simulink model "CSE1_CV3_1Straight"  (Simulink 7.3)
settings: Solver=ode4  StartTime=0.0  StopTime=inf  FixedStep=0.1  RelTol=1e-3
undefined symbols (not defined in the file or in its folder): eta1_0_real, v1_0_real, velocitySatValues1
libraries: simulink x68, dspmtrx3 x24, simulink_extras x23, marine_gnc x5, dspindex x5, dspinverses x4
(part 2 of 6)

== system CSE1_CV3_1Straight/Plants/CSE1 ==
  Thurster setting : Inport
  Enable : EnablePort  StatesWhenEnabling=reset
  Bow Thruster : Subsystem
  Demux : Demux  Outputs=7
  "Voith Schneider Propeller " : Subsystem
  wires:
  Thurster setting/1 -> Demux/1
  Demux/1 -> "Voith Schneider Propeller "/1(Port VSP y u_1)
  Demux/2 -> "Voith Schneider Propeller "/2(Port VSP x u_2)
  Demux/3 -> "Voith Schneider Propeller "/3(Starboard VSP y u_3)
  Demux/4 -> "Voith Schneider Propeller "/4(Starboard VSP x u_4)
  Demux/7 -> "Voith Schneider Propeller "/5(VSP Speed)
  Demux/5 -> Bow Thruster/1(Bow Thruster Direction u_5)
  Demux/6 -> Bow Thruster/2(Bow Thruster Power)

== system CSE1_CV3_1Straight/Plants/Linear Simulator ==
  tau : Inport
  Enable : EnablePort  StatesWhenEnabling=reset
  Demux1 : Demux  Outputs=3
  Demux2 : Demux  Outputs=3
  Demux3 : Demux  Outputs=3
  Linear Vessel Dynamics : Subsystem
  Mux1 : Mux  Inputs=3
  Mux2 : Mux  Inputs=3
  Mux3 : Mux  Inputs=3
  eta_surge_hil : Gain  ParameterDataType=fixdt(1, 16)  ParameterScaling=2^0  OutDataType=fixdt(1, 16)  OutScaling=2^0
  eta_sway_hil : Gain  ParameterDataType=fixdt(1, 16)  ParameterScaling=2^0  OutDataType=fixdt(1, 16)  OutScaling=2^0
  eta_yaw_hil : Gain  ParameterDataType=fixdt(1, 16)  ParameterScaling=2^0  OutDataType=fixdt(1, 16)  OutScaling=2^0
  etadot : Terminator
  etadot_surge_hil : Gain  ParameterDataType=fixdt(1, 16)  ParameterScaling=2^0  OutDataType=fixdt(1, 16)  OutScaling=2^0
  etadot_sway_hil : Gain  ParameterDataType=fixdt(1, 16)  ParameterScaling=2^0  OutDataType=fixdt(1, 16)  OutScaling=2^0
  etadot_yaw_hil : Gain  ParameterDataType=fixdt(1, 16)  ParameterScaling=2^0  OutDataType=fixdt(1, 16)  OutScaling=2^0
  nu_surge_hil : Gain  ParameterDataType=fixdt(1, 16)  ParameterScaling=2^0  OutDataType=fixdt(1, 16)  OutScaling=2^0
  nu_sway_hil : Gain  ParameterDataType=fixdt(1, 16)  ParameterScaling=2^0  OutDataType=fixdt(1, 16)  OutScaling=2^0
  nu_yaw_hil : Gain  ParameterDataType=fixdt(1, 16)  ParameterScaling=2^0  OutDataType=fixdt(1, 16)  OutScaling=2^0
  eta_hil : Outport
  nu_hil : Outport  Port=2
  wires:
  nu_yaw_hil/1 -> Mux1/3
  nu_sway_hil/1 -> Mux1/2
  nu_surge_hil/1 -> Mux1/1
  Demux2/3 -> nu_yaw_hil/1
  Demux2/2 -> nu_sway_hil/1
  Demux2/1 -> nu_surge_hil/1
  eta_sway_hil/1 -> Mux3/2
  eta_yaw_hil/1 -> Mux3/3
  eta_surge_hil/1 -> Mux3/1
  Demux1/3 -> eta_yaw_hil/1
  Demux1/2 -> eta_sway_hil/1
  Demux1/1 -> eta_surge_hil/1
  Linear Vessel Dynamics/1(eta) -> Demux1/1
  Linear Vessel Dynamics/2(nu) -> Demux2/1
  Mux1/1 -> nu_hil/1
  Mux3/1 -> eta_hil/1
  etadot_sway_hil/1 -> Mux2/2
  etadot_yaw_hil/1 -> Mux2/3
  etadot_surge_hil/1 -> Mux2/1
  Demux3/3 -> etadot_yaw_hil/1
  Demux3/2 -> etadot_sway_hil/1
  Demux3/1 -> etadot_surge_hil/1
  Linear Vessel Dynamics/3(etadot) -> Demux3/1
  Mux2/1 -> etadot/1
  tau/1 -> Linear Vessel Dynamics/1(tau)

== system CSE1_CV3_1Straight/Plants/saturation ==
  tau : Inport  OutDataType=sfix(16)  OutScaling=2^0
  Demux : Demux  Outputs=3
  Mux1 : Mux  Inputs=3
  Saturation : Saturate  UpperLimit=3  LowerLimit=-2.6
  Saturation1 : Saturate  UpperLimit=3  LowerLimit=-3.5
  Saturation2 : Saturate  UpperLimit=1.6  LowerLimit=-1.5
  plant tau_surge : Gain  ParameterDataType=fixdt(1, 16)  ParameterScaling=2^0  OutDataType=fixdt(1, 16)  OutScaling=2^0
  plant tau_sway : Gain  ParameterDataType=fixdt(1, 16)  ParameterScaling=2^0  OutDataType=fixdt(1, 16)  OutScaling=2^0
  plant tau_yaw : Gain  ParameterDataType=fixdt(1, 16)  ParameterScaling=2^0  OutDataType=fixdt(1, 16)  OutScaling=2^0
  sat_tau : Outport  OutDataType=sfix(16)  OutScaling=2^0
  wires:
  Saturation2/1 -> plant tau_yaw/1
  Saturation1/1 -> plant tau_sway/1
  Saturation/1 -> plant tau_surge/1
  Demux/3 -> Saturation2/1
  Demux/2 -> Saturation1/1
  Demux/1 -> Saturation/1
  tau/1 -> Demux/1
  Mux1/1 -> sat_tau/1
  plant tau_surge/1 -> Mux1/1
  plant tau_sway/1 -> Mux1/2
  plant tau_yaw/1 -> Mux1/3

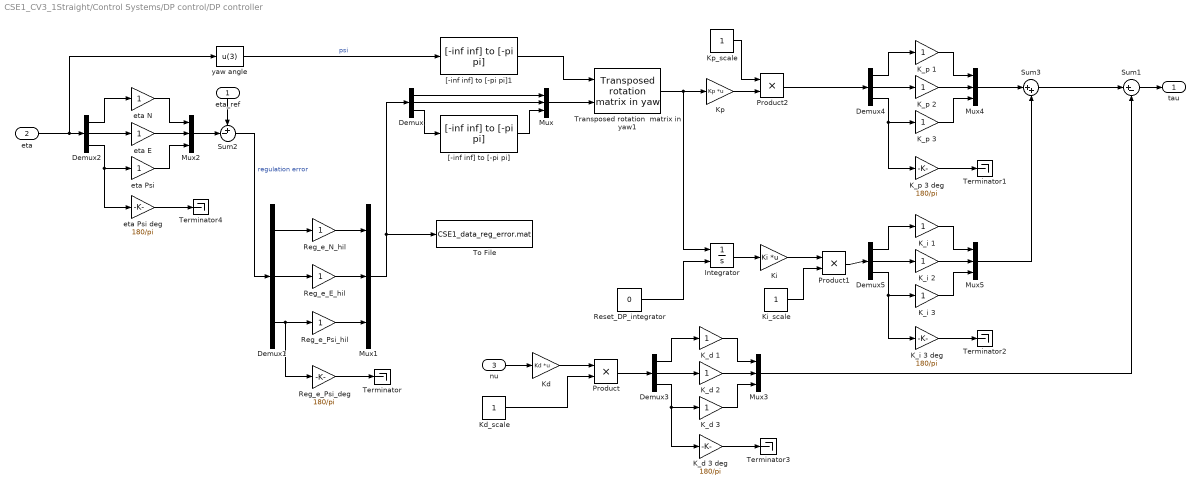
== system CSE1_CV3_1Straight/Control Systems/DP control/DP controller ==
  eta_ref : Inport
  eta : Inport  Port=2
  nu : Inport  Port=3
  Demux{,1..5} (6 alike) : Demux  Outputs=3
  Integrator : Integrator  ExternalReset=level
  K_d 1 : Gain  ParameterDataType=fixdt(1, 16)  ParameterScaling=2^0  OutDataType=fixdt(1, 16)  OutScaling=2^0
  K_d 2 : Gain  ParameterDataType=fixdt(1, 16)  ParameterScaling=2^0  OutDataType=fixdt(1, 16)  OutScaling=2^0
  K_d 3 : Gain  ParameterDataType=fixdt(1, 16)  ParameterScaling=2^0  OutDataType=fixdt(1, 16)  OutScaling=2^0
  K_d 3 deg : Gain  Gain=180/pi  ParameterDataType=fixdt(1, 16)  ParameterScaling=2^0  OutDataType=fixdt(1, 16)  OutScaling=2^0
  K_i 1 : Gain  ParameterDataType=fixdt(1, 16)  ParameterScaling=2^0  OutDataType=fixdt(1, 16)  OutScaling=2^0
  K_i 2 : Gain  ParameterDataType=fixdt(1, 16)  ParameterScaling=2^0  OutDataType=fixdt(1, 16)  OutScaling=2^0
  K_i 3 : Gain  ParameterDataType=fixdt(1, 16)  ParameterScaling=2^0  OutDataType=fixdt(1, 16)  OutScaling=2^0
  K_i 3 deg : Gain  Gain=180/pi  ParameterDataType=fixdt(1, 16)  ParameterScaling=2^0  OutDataType=fixdt(1, 16)  OutScaling=2^0
  K_p 1 : Gain  ParameterDataType=fixdt(1, 16)  ParameterScaling=2^0  OutDataType=fixdt(1, 16)  OutScaling=2^0
  K_p 2 : Gain  ParameterDataType=fixdt(1, 16)  ParameterScaling=2^0  OutDataType=fixdt(1, 16)  OutScaling=2^0
  K_p 3 : Gain  ParameterDataType=fixdt(1, 16)  ParameterScaling=2^0  OutDataType=fixdt(1, 16)  OutScaling=2^0
  K_p 3 deg : Gain  Gain=180/pi  ParameterDataType=fixdt(1, 16)  ParameterScaling=2^0  OutDataType=fixdt(1, 16)  OutScaling=2^0
  Kd : Gain  Gain=Kd  Multiplication=Matrix(K*u)  SaturateOnIntegerOverflow=on  OutDataTypeStr=Inherit: Same as input  ParamDataTypeStr=Inherit: Same as input
  Kd_scale : Constant
  Ki : Gain  Gain=Ki  Multiplication=Matrix(K*u)  SaturateOnIntegerOverflow=on  OutDataTypeStr=Inherit: Same as input  ParamDataTypeStr=Inherit: Same as input
  Ki_scale : Constant
  Kp : Gain  Gain=Kp  Multiplication=Matrix(K*u)  SaturateOnIntegerOverflow=on  OutDataTypeStr=Inherit: Same as input  ParamDataTypeStr=Inherit: Same as input
  Kp_scale : Constant
  Mux{,1..5} (6 alike) : Mux  Inputs=3
  Product : Product  RndMeth=Zero
  Product1 : Product  RndMeth=Zero
  Product2 : Product  RndMeth=Zero
  Reg_e_E_hil : Gain
  Reg_e_N_hil : Gain
  Reg_e_Psi_deg : Gain  Gain=180/pi  ParameterDataType=fixdt(1, 16)  ParameterScaling=2^0  OutDataType=fixdt(1, 16)  OutScaling=2^0
  Reg_e_Psi_hil : Gain
  Reset_DP_integrator : Constant  Value=0
  Sum1 : Sum  Inputs=|+-  SaturateOnIntegerOverflow=on  InputSameDT=on  OutDataTypeStr=Inherit: Same as first input
  Sum2 : Sum  Inputs=+-|  SaturateOnIntegerOverflow=on  InputSameDT=on  OutDataTypeStr=Inherit: Same as first input
  Sum3 : Sum  Inputs=|++  SaturateOnIntegerOverflow=on  InputSameDT=on  OutDataTypeStr=Inherit: Same as first input
  Terminator{,1..4} (5 alike) : Terminator
  To File : ToFile  Filename=CSE1_data_reg_error.mat  MatrixName=cse1_data_reg_error
  Transposed rotation  matrix in yaw1 : marine_gnc/Models/ Kinematics/Transposed rotation  matrix in yaw  SystemSampleTime=-1
  "[-inf inf] to [-pi pi]" : marine_gnc/Utilities/Math Operations/[-inf inf] to [-pi pi]  SystemSampleTime=-1
  "[-inf inf] to [-pi pi]1" : marine_gnc/Utilities/Math Operations/[-inf inf] to [-pi pi]  SystemSampleTime=-1
  eta E : Gain  ParameterDataType=fixdt(1, 16)  ParameterScaling=2^0  OutDataType=fixdt(1, 16)  OutScaling=2^0
  eta N : Gain  ParameterDataType=fixdt(1, 16)  ParameterScaling=2^0  OutDataType=fixdt(1, 16)  OutScaling=2^0
  eta Psi : Gain  ParameterDataType=fixdt(1, 16)  ParameterScaling=2^0  OutDataType=fixdt(1, 16)  OutScaling=2^0
  eta Psi deg : Gain  Gain=180/pi  ParameterDataType=fixdt(1, 16)  ParameterScaling=2^0  OutDataType=fixdt(1, 16)  OutScaling=2^0
  yaw angle : Fcn  Expr=u(3)
  tau : Outport  InitialOutput=0
  wires:
  Mux/1 -> Transposed rotation  matrix in yaw1/2
  Demux/1 -> Mux/1
  Demux/2 -> Mux/2
  eta_ref/1 -> Sum2/1
  Sum1/1 -> tau/1
  eta/1 -> yaw angle/1, Demux2/1
  Integrator/1 -> Ki/1
  Sum3/1 -> Sum1/1
  Transposed rotation  matrix in yaw1/1 -> Kp/1, Integrator/1
  Demux1/1 -> Reg_e_N_hil/1
  Reg_e_N_hil/1 -> Mux1/1
  Sum2/1 -> Demux1/1  "regulation error"
  Demux1/2 -> Reg_e_E_hil/1
  Reg_e_E_hil/1 -> Mux1/2
  Demux1/3 -> Reg_e_Psi_hil/1, Reg_e_Psi_deg/1
  Reg_e_Psi_hil/1 -> Mux1/3
  Mux1/1 -> Demux/1, To File/1
  nu/1 -> Kd/1
  Kd/1 -> Product/1
  Kd_scale/1 -> Product/2
  Ki/1 -> Product1/1
  Ki_scale/1 -> Product1/2
  Kp/1 -> Product2/2
  Kp_scale/1 -> Product2/1
  Reset_DP_integrator/1 -> Integrator/2
  yaw angle/1 -> "[-inf inf] to [-pi pi]1"/1  "psi"
  "[-inf inf] to [-pi pi]1"/1 -> Transposed rotation  matrix in yaw1/1
  Demux/3 -> "[-inf inf] to [-pi pi]"/1
  "[-inf inf] to [-pi pi]"/1 -> Mux/3
  eta N/1 -> Mux2/1
  eta E/1 -> Mux2/2
  eta Psi/1 -> Mux2/3
  Demux2/1 -> eta N/1
  Demux2/2 -> eta E/1
  Demux2/3 -> eta Psi/1, eta Psi deg/1
  Mux2/1 -> Sum2/2
  K_d 1/1 -> Mux3/1
  K_d 2/1 -> Mux3/2
  K_d 3/1 -> Mux3/3
  Demux3/1 -> K_d 1/1
  Demux3/2 -> K_d 2/1
  Demux3/3 -> K_d 3/1, K_d 3 deg/1
  Product/1 -> Demux3/1
  Mux3/1 -> Sum1/2
  K_p 1/1 -> Mux4/1
  K_p 2/1 -> Mux4/2
  K_p 3/1 -> Mux4/3
  Demux4/1 -> K_p 1/1
  Demux4/2 -> K_p 2/1
  Demux4/3 -> K_p 3/1, K_p 3 deg/1
  Product2/1 -> Demux4/1
  Mux4/1 -> Sum3/1
  K_i 1/1 -> Mux5/1
  K_i 2/1 -> Mux5/2
  K_i 3/1 -> Mux5/3
  Demux5/1 -> K_i 1/1
  Demux5/2 -> K_i 2/1
  Demux5/3 -> K_i 3/1, K_i 3 deg/1
  Product1/1 -> Demux5/1
  Mux5/1 -> Sum3/2
  K_p 3 deg/1 -> Terminator1/1
  K_i 3 deg/1 -> Terminator2/1
  K_d 3 deg/1 -> Terminator3/1
  Reg_e_Psi_deg/1 -> Terminator/1
  eta Psi deg/1 -> Terminator4/1

== system CSE1_CV3_1Straight/Control Systems/DP control/Thruster allocation ==
  tau : Inport
  f_act to u_act : Subsystem
  tau to f_act : Subsystem
  u_act : Outport
  wires:
  tau/1 -> tau to f_act/1(tau)
  tau to f_act/1(f_act) -> f_act to u_act/1(f_act)
  f_act to u_act/1(u_act) -> u_act/1

== system CSE1_CV3_1Straight/Control Systems/LgV design 2/Auxilary functions g_q ==
  f_q : Inport
  psi_los^q : Inport  Port=2
  f_q^q : Inport  Port=3
  psi_los^q^2 : Inport  Port=4
  f_q^s : Inport  Port=5
  psi_los^qs : Inport  Port=6
  f_q^t : Inport  Port=7
  g_q eq : Subsystem
  g_q^q eq : Subsystem
  g_q^s eq : Subsystem
  g_q^t eq : Subsystem
  g_q : Outport
  g_q^t : Outport  Port=2
  g_q^q : Outport  Port=3
  g_q^s : Outport  Port=4
  wires:
  g_q eq/1(g_q) -> g_q/1
  psi_los^q/1 -> g_q eq/2(psi_los^q), g_q^q eq/2(psi_los^q), g_q^s eq/2(psi_los^q), g_q^t eq/1(psi_los^q)
  f_q/1 -> g_q eq/1(f_q), g_q^q eq/1(f_q), g_q^s eq/1(f_q)
  f_q^q/1 -> g_q^q eq/3(f_q^q)
  psi_los^q^2/1 -> g_q^q eq/4(psi_los^q^2)
  g_q^q eq/1(g_q^q) -> g_q^q/1
  g_q^s eq/1(g_q^s) -> g_q^s/1
  f_q^s/1 -> g_q^s eq/3(f_q^s)
  psi_los^qs/1 -> g_q^s eq/4(psi_los^qs)
  g_q^t eq/1(g_q^t) -> g_q^t/1
  f_q^t/1 -> g_q^t eq/2(f_q^t)

== system CSE1_CV3_1Straight/Control Systems/LgV design 2/Auxiliary function g_s ==
  psi_los^sq : Inport
  f_s : Inport  Port=2
  psi_los^s : Inport  Port=3
  f_s^q : Inport  Port=4
  f_s^s : Inport  Port=5
  psi_los^s^2 : Inport  Port=6
  f_s^t : Inport  Port=7
  g_s eq : Subsystem
  g_s^q eq : Subsystem
  g_s^s eq : Subsystem
  g_s^t eq : Subsystem
  g_s^q : Outport
  g_s^s : Outport  Port=2
  g_s^t : Outport  Port=3
  g_s : Outport  Port=4
  wires:
  f_s/1 -> g_s eq/1(f_s), g_s^q eq/1(f_s), g_s^s eq/1(f_s)
  psi_los^s/1 -> g_s eq/2(psi_los^s), g_s^q eq/2(psi_los^s), g_s^s eq/2(psi_los^s), g_s^t eq/1(psi_los^s)
  g_s eq/1(g_s) -> g_s/1
  f_s^q/1 -> g_s^q eq/3(f_s^q)
  psi_los^sq/1 -> g_s^q eq/4(psi_los^sq)
  g_s^q eq/1(g_s^q) -> g_s^q/1
  g_s^s eq/1(g_s^s) -> g_s^s/1
  f_s^s/1 -> g_s^s eq/3(f_s^s)
  psi_los^s^2/1 -> g_s^s eq/4(psi_los^s^2)
  g_s^t eq/1(g_a^t) -> g_s^t/1
  f_s^t/1 -> g_s^t eq/2(f_s^t)

== system CSE1_CV3_1Straight/Control Systems/LgV design 2/Control law ==
  R^T : Inport
  kappa1 : Inport  Port=2
  sigma : Inport  Port=3
  alpha^q : Inport  Port=4
  alpha^s : Inport  Port=5
  nu : Inport  Port=6
  z_2 : Inport  Port=7
  zeta : Inport  Port=8
  omega_q : Inport  Port=9
  K_i : Inport  Port=10
  K_d : Inport  Port=11
  M : Inport  Port=12
  f_q : Inport  Port=13
  f_s : Inport  Port=14
  1 : Constant  OutDataType=fixdt(1, 16)  OutScaling=2^0
  4 : Gain  Gain=4  ParameterDataType=fixdt(1, 16)  ParameterScaling=2^0  OutDataType=fixdt(1, 16)  OutScaling=2^0
  Add1 : Sum  OutDataType=fixdt(1, 16)  OutScaling=2^-10
  Add2 : Sum  OutDataType=fixdt(1, 16)  OutScaling=2^-10
  D_L : Subsystem
  Divide : Product  Inputs=*/  OutDataType=fixdt(1, 16)  OutScaling=2^-10
  Product : Product  Inputs=3  Multiplication=Matrix(*)  OutDataType=fixdt(1, 16)  OutScaling=2^0  RndMeth=Zero
  Product1 : Product  Multiplication=Matrix(*)  OutDataType=fixdt(1, 16)  OutScaling=2^0  RndMeth=Zero
  Product2 : Product  Multiplication=Matrix(*)  OutDataType=fixdt(1, 16)  OutScaling=2^0  RndMeth=Zero
  Product4 : Product  Multiplication=Matrix(*)  OutDataType=fixdt(1, 16)  OutScaling=2^0  RndMeth=Zero
  Product5 : Product  Inputs=3  Multiplication=Matrix(*)  OutDataType=fixdt(1, 16)  OutScaling=2^0  RndMeth=Zero
  Product6 : Product  Inputs=3  Multiplication=Matrix(*)  OutDataType=fixdt(1, 16)  OutScaling=2^0  RndMeth=Zero
  Sum : Sum  Inputs=--++++  OutDataType=fixdt(1, 16)  OutScaling=2^-10
  tau : Outport
  wires:
  Sum/1 -> tau/1
  R^T/1 -> Product/1
  K_i/1 -> Product/2
  zeta/1 -> Product/3
  K_d/1 -> Add1/1
  Divide/1 -> Add1/2
  1/1 -> Divide/1
  kappa1/1 -> 4/1
  4/1 -> Divide/2
  Add1/1 -> Product1/1
  z_2/1 -> Product1/2
  Product1/1 -> Sum/2
  nu/1 -> Product2/2
  D_L/1(D_L) -> Product2/1
  Product2/1 -> Sum/3
  M/1 -> Product4/1, Product5/1, Product6/1
  sigma/1 -> Product4/2
  Product4/1 -> Sum/4
  alpha^q/1 -> Product5/2
  Product5/1 -> Sum/5
  alpha^s/1 -> Product6/2
  f_s/1 -> Product6/3
  Product6/1 -> Sum/6
  omega_q/1 -> Add2/1
  f_q/1 -> Add2/2
  Add2/1 -> Product5/3
  Product/1 -> Sum/1

== system CSE1_CV3_1Straight/Control Systems/LgV design 2/Gamma_q ==
  11 : Inport
  22 : Inport  Port=2
  12 : Constant  Value=0
  21 : Constant  Value=0
  2x2 : Reshape  OutputDimensionality=Customize  OutputDimensions=[2,2]
  Mux : Mux
  Gamma_q : Outport
  wires:
  2x2/1 -> Gamma_q/1
  Mux/1 -> 2x2/1
  11/1 -> Mux/1
  21/1 -> Mux/2
  12/1 -> Mux/3
  22/1 -> Mux/4

== system CSE1_CV3_1Straight/Control Systems/LgV design 2/Integral action state ==
  z_2 : Inport
  R : Inport  Port=2
  Integrator : Integrator  InitialCondition=[0 0 0]'
  Product : Product  Multiplication=Matrix(*)  OutDataType=fixdt(1, 16)  OutScaling=2^0  RndMeth=Zero
  zeta : Outport
  wires:
  R/1 -> Product/1
  z_2/1 -> Product/2
  Integrator/1 -> zeta/1
  Product/1 -> Integrator/1

== system CSE1_CV3_1Straight/Control Systems/LgV design 2/K_d ==
  11 : Inport
  22 : Inport  Port=2
  33 : Inport  Port=3
  {12..13,21,23,31..32} (6 alike) : Constant  Value=0
  3x3 : Reshape  OutputDimensionality=Customize  OutputDimensions=[3,3]
  Mux : Mux  Inputs=9
  K_d : Outport
  wires:
  3x3/1 -> K_d/1
  Mux/1 -> 3x3/1
  11/1 -> Mux/1
  21/1 -> Mux/2
  31/1 -> Mux/3
  12/1 -> Mux/4
  22/1 -> Mux/5
  32/1 -> Mux/6
  13/1 -> Mux/7
  23/1 -> Mux/8
  33/1 -> Mux/9

== system CSE1_CV3_1Straight/Control Systems/LgV design 2/K_i ==
  11 : Inport
  22 : Inport  Port=2
  33 : Inport  Port=3
  {12..13,21,23,31..32} (6 alike) : Constant  Value=0
  3x3 : Reshape  OutputDimensionality=Customize  OutputDimensions=[3,3]
  Mux : Mux  Inputs=9
  K_i : Outport
  wires:
  3x3/1 -> K_i/1
  Mux/1 -> 3x3/1
  11/1 -> Mux/1
  21/1 -> Mux/2
  31/1 -> Mux/3
  12/1 -> Mux/4
  22/1 -> Mux/5
  32/1 -> Mux/6
  13/1 -> Mux/7
  23/1 -> Mux/8
  33/1 -> Mux/9

== system CSE1_CV3_1Straight/Control Systems/LgV design 2/K_p ==
  11 : Inport
  22 : Inport  Port=2
  33 : Inport  Port=3
  {12..13,21,23,31..32} (6 alike) : Constant  Value=0
  Mux : Mux  Inputs=9
  R(psi) : Reshape  OutputDimensionality=Customize  OutputDimensions=[3,3]
  K_p : Outport
  wires:
  R(psi)/1 -> K_p/1
  Mux/1 -> R(psi)/1
  11/1 -> Mux/1
  21/1 -> Mux/2
  31/1 -> Mux/3
  12/1 -> Mux/4
  22/1 -> Mux/5
  32/1 -> Mux/6
  13/1 -> Mux/7
  23/1 -> Mux/8
  33/1 -> Mux/9

== system CSE1_CV3_1Straight/Control Systems/LgV design 2/M ==
  3x3 : Reshape  OutputDimensionality=Customize  OutputDimensions=[3,3]
  I_z : Constant  Value=1.760
  M_{11,22..23,32..33} (5 alike) : Sum  Inputs=+-
  M_{12..13,21,31} (4 alike) : Constant  Value=0
  Mux : Mux  Inputs=9
  N_rdot : Constant  Value=-1.0
  N_vdot : Constant  Value=-0.0
  X_udot : Constant  Value=-2.0
  Y_rdot : Constant  Value=0.0
  Y_vdot : Constant  Value=-10.0
  m : Constant  Value=17.6
  m x_g : Product  RndMeth=Zero
  x_g : Constant  Value=0.03
  M : Outport
  wires:
  3x3/1 -> M/1
  Mux/1 -> 3x3/1
  M_33/1 -> Mux/9
  M_23/1 -> Mux/8
  M_13/1 -> Mux/7
  M_32/1 -> Mux/6
  M_22/1 -> Mux/5
  M_12/1 -> Mux/4
  M_31/1 -> Mux/3
  M_21/1 -> Mux/2
  M_11/1 -> Mux/1
  N_rdot/1 -> M_33/2
  I_z/1 -> M_33/1
  Y_rdot/1 -> M_23/2
  N_vdot/1 -> M_32/2
  m x_g/1 -> M_23/1, M_32/1
  x_g/1 -> m x_g/2
  Y_vdot/1 -> M_22/2
  X_udot/1 -> M_11/2
  m/1 -> m x_g/1, M_22/1, M_11/1

== system CSE1_CV3_1Straight/Control Systems/LgV design 2/R(psi) ==
  psi : Inport
  -1 : Gain  Gain=-1  ParameterDataType=fixdt(1, 16)  ParameterScaling=2^0  OutDataType=fixdt(1, 16)  OutScaling=2^0
  Mux : Mux  Inputs=9
  R(psi) : Reshape  OutputDimensionality=Customize  OutputDimensions=[3,3]
  R11 : Trigonometry  Operator=cos
  R12 : Trigonometry
  R{13,23,31..32} (4 alike) : Constant  Value=0
  R21 : Trigonometry
  R22 : Trigonometry  Operator=cos
  R33 : Constant
  R : Outport
  wires:
  R(psi)/1 -> R/1
  Mux/1 -> R(psi)/1
  psi/1 -> R11/1, R21/1, R12/1, R22/1
  R11/1 -> Mux/1
  R21/1 -> Mux/2
  R31/1 -> Mux/3
  R12/1 -> -1/1
  R22/1 -> Mux/5
  R32/1 -> Mux/6
  R13/1 -> Mux/7
  R33/1 -> Mux/9
  R23/1 -> Mux/8
  -1/1 -> Mux/4

== system CSE1_CV3_1Straight/Control Systems/LgV design 2/S(r) ==
  r : Inport
  Mux : Mux  Inputs=9
  R31 : Constant  Value=0
  S(r) : Reshape  OutputDimensionality=Customize  OutputDimensions=[3,3]
  S{11,13,22..23,32} (5 alike) : Constant  Value=0
  S12 : Gain  ParameterDataType=fixdt(1, 16)  ParameterScaling=2^0  OutDataType=fixdt(1, 16)  OutScaling=2^0
  S33 : Constant
  S : Outport
  wires:
  S(r)/1 -> S/1
  Mux/1 -> S(r)/1
  R31/1 -> Mux/3
  S12/1 -> Mux/4
  S22/1 -> Mux/5
  S32/1 -> Mux/6
  S13/1 -> Mux/7
  S33/1 -> Mux/9
  S23/1 -> Mux/8
  r/1 -> Mux/2, S12/1
  S11/1 -> Mux/1

== system CSE1_CV3_1Straight/Control Systems/LgV design 2/Thruster allocation ==
  tau : Inport
  f_act to u_act : Subsystem
  tau to f_act : Subsystem
  u_act : Outport
  wires:
  tau/1 -> tau to f_act/1(tau)
  tau to f_act/1(f_act) -> f_act to u_act/1(f_act)
  f_act to u_act/1(u_act) -> u_act/1

== system CSE1_CV3_1Straight/Control Systems/LgV design 2/Update laws ==
  V_1^q : Inport
  Gamma_q : Inport  Port=2
  lambda : Inport  Port=3
  f_q : Inport  Port=4
  f_s : Inport  Port=5
  Add : Sum  OutDataType=fixdt(1, 16)  OutScaling=2^-10
  Add1 : Sum  OutDataType=fixdt(1, 16)  OutScaling=2^-10
  Gain : Gain  Gain=-1  ParameterDataType=fixdt(1, 16)  ParameterScaling=2^0  OutDataType=fixdt(1, 16)  OutScaling=2^0
  Integrator : Integrator  ExternalReset=level  InitialConditionSource=external
  Integrator1 : Integrator  ExternalReset=level  InitialConditionSource=external  InitialCondition=250
  Integrator2 : Integrator
  Product : Product  Multiplication=Matrix(*)  OutDataType=fixdt(1, 16)  OutScaling=2^0  RndMeth=Zero
  Product1 : Product  OutDataType=fixdt(1, 16)  OutScaling=2^0  RndMeth=Zero
  Reset q : Constant  Value=0
  Reset s : Constant  Value=0
  Transpose : dspmtrx3/Transpose  SystemSampleTime=-1  Hermitian=off  overflowFlag=off
  q_0 : Subsystem
  s_0 : Constant  Value=0
  omega_q : Outport
  q : Outport  Port=2  PortDimensions=2
  s : Outport  Port=3  PortDimensions=1
  wires:
  f_q/1 -> Add/2
  Add/1 -> Integrator/1
  Product/1 -> Add1/2
  V_1^q/1 -> Transpose/1
  Gamma_q/1 -> Product/1
  lambda/1 -> Product1/1
  Add1/1 -> Product1/2
  Product1/1 -> Gain/1
  Gain/1 -> Integrator2/1
  f_s/1 -> Integrator1/1
  Transpose/1 -> Product/2
  Integrator/1 -> q/1
  Integrator1/1 -> s/1
  Integrator2/1 -> omega_q/1, Add/1, Add1/1
  Reset s/1 -> Integrator1/2
  s_0/1 -> Integrator1/3
  Reset q/1 -> Integrator/2
  q_0/1(q_0) -> Integrator/3

== system CSE1_CV3_1Straight/Control Systems/LgV design 2/V_1^q ==
  chi^q : Inport
  z_1 : Inport  Port=2
  R^T : Inport  Port=3
  Gain : Gain  Gain=-1  ParameterDataType=fixdt(1, 16)  ParameterScaling=2^0  OutDataType=fixdt(1, 16)  OutScaling=2^0
  Product : Product  Inputs=3  Multiplication=Matrix(*)  OutDataType=fixdt(1, 16)  OutScaling=2^0  RndMeth=Zero
  Transpose : dspmtrx3/Transpose  SystemSampleTime=-1  Hermitian=off  overflowFlag=off
  V_1^q : Outport
  wires:
  Product/1 -> Gain/1
  R^T/1 -> Product/2
  z_1/1 -> Transpose/1
  Transpose/1 -> Product/1
  chi^q/1 -> Product/3
  Gain/1 -> V_1^q/1

== system CSE1_CV3_1Straight/Control Systems/LgV design 2/Virtual control ==
  g_q : Inport
  g_s : Inport  Port=2
  K_p : Inport  Port=3
  kappa_1 : Inport  Port=4
  R^T : Inport  Port=5
  z_1 : Inport  Port=6
  Add : Sum  OutDataType=fixdt(1, 16)  OutScaling=2^-10
  I : dspmtrx3/Constant Diagonal Matrix  SystemSampleTime=-1  q=[1 1 1 ]  frame=off  dataType=Inherit from 'Constant(s) along diagonal'  isSigned=on  wordLen=16  udDataType=sfix(16)  fracBitsMode=Best precision  numFracBits=15
  Product : Product  OutDataType=fixdt(1, 16)  OutScaling=2^0  RndMeth=Zero
  Product1 : Product  Multiplication=Matrix(*)  OutDataType=fixdt(1, 16)  OutScaling=2^0  RndMeth=Zero
  Product2 : Product  Multiplication=Matrix(*)  OutDataType=fixdt(1, 16)  OutScaling=2^0  RndMeth=Zero
  Subtract : Sum  Inputs=+-  OutDataType=fixdt(1, 16)  OutScaling=2^-10
  Sum : Sum  Inputs=-+  OutDataType=fixdt(1, 16)  OutScaling=2^-10
  alpha : Outport
  wires:
  Sum/1 -> alpha/1
  K_p/1 -> Subtract/1
  kappa_1/1 -> Product/1
  I/1 -> Product/2
  Product/1 -> Subtract/2
  Subtract/1 -> Product1/1
  z_1/1 -> Product1/2
  Product1/1 -> Sum/1
  R^T/1 -> Product2/1
  g_q/1 -> Add/1
  g_s/1 -> Add/2
  Add/1 -> Product2/2
  Product2/1 -> Sum/2

== system CSE1_CV3_1Straight/Control Systems/LgV design 2/alpha^q ==
  kappa1 : Inport
  R^T : Inport  Port=2
  K_p : Inport  Port=3
  g_q^q : Inport  Port=4
  g_s^q : Inport  Port=5
  chi^q : Inport  Port=6
  Add2 : Sum  OutDataType=fixdt(1, 16)  OutScaling=2^-10
  Add3 : Sum  OutDataType=fixdt(1, 16)  OutScaling=2^-10
  I : dspmtrx3/Constant Diagonal Matrix  SystemSampleTime=-1  q=[1 1 1 ]  frame=off  dataType=Inherit from 'Constant(s) along diagonal'  isSigned=on  wordLen=16  udDataType=sfix(16)  fracBitsMode=Best precision  numFracBits=15
  Product1 : Product  OutDataType=fixdt(1, 16)  OutScaling=2^0  RndMeth=Zero
  Product3 : Product  Inputs=3  Multiplication=Matrix(*)  OutDataType=fixdt(1, 16)  OutScaling=2^0  RndMeth=Zero
  Product4 : Product  Multiplication=Matrix(*)  OutDataType=fixdt(1, 16)  OutScaling=2^0  RndMeth=Zero
  Subtract : Sum  Inputs=+-  OutDataType=fixdt(1, 16)  OutScaling=2^-10
  alpha^q : Outport
  wires:
  Add3/1 -> alpha^q/1
  K_p/1 -> Subtract/1
  Product1/1 -> Subtract/2
  kappa1/1 -> Product1/1
  I/1 -> Product1/2
  Subtract/1 -> Product3/1
  g_q^q/1 -> Add2/1
  g_s^q/1 -> Add2/2
  Add2/1 -> Product4/2
  R^T/1 -> Product3/2, Product4/1
  chi^q/1 -> Product3/3
  Product3/1 -> Add3/1
  Product4/1 -> Add3/2

== system CSE1_CV3_1Straight/Control Systems/LgV design 2/alpha^s ==
  kappa1 : Inport
  R^T : Inport  Port=2
  K_p : Inport  Port=3
  g_q^s : Inport  Port=4
  g_s^s : Inport  Port=5
  chi^s : Inport  Port=6
  Add2 : Sum  OutDataType=fixdt(1, 16)  OutScaling=2^-10
  Add3 : Sum  OutDataType=fixdt(1, 16)  OutScaling=2^-10
  I : dspmtrx3/Constant Diagonal Matrix  SystemSampleTime=-1  q=[1 1 1 ]  frame=off  dataType=Inherit from 'Constant(s) along diagonal'  isSigned=on  wordLen=16  udDataType=sfix(16)  fracBitsMode=Best precision  numFracBits=15
  Product1 : Product  OutDataType=fixdt(1, 16)  OutScaling=2^0  RndMeth=Zero
  Product3 : Product  Inputs=3  Multiplication=Matrix(*)  OutDataType=fixdt(1, 16)  OutScaling=2^0  RndMeth=Zero
  Product4 : Product  Multiplication=Matrix(*)  OutDataType=fixdt(1, 16)  OutScaling=2^0  RndMeth=Zero
  Subtract : Sum  Inputs=+-  OutDataType=fixdt(1, 16)  OutScaling=2^-10
  alpha^s : Outport
  wires:
  Add3/1 -> alpha^s/1
  K_p/1 -> Subtract/1
  Product1/1 -> Subtract/2
  kappa1/1 -> Product1/1
  I/1 -> Product1/2
  Subtract/1 -> Product3/1
  g_q^s/1 -> Add2/1
  g_s^s/1 -> Add2/2
  Add2/1 -> Product4/2
  R^T/1 -> Product3/2, Product4/1
  chi^s/1 -> Product3/3
  Product3/1 -> Add3/1
  Product4/1 -> Add3/2

== system CSE1_CV3_1Straight/Control Systems/LgV design 2/sigma eq ==
  kappa1 : Inport
  R^T : Inport  Port=2
  K_p : Inport  Port=3
  S^T : Inport  Port=4
  g_q : Inport  Port=5
  nu : Inport  Port=6
  g_q^t : Inport  Port=7
  g_s : Inport  Port=8
  g_s^t : Inport  Port=9
  z_1 : Inport  Port=10
  Add : Sum  OutDataType=fixdt(1, 16)  OutScaling=2^-10
  Add1 : Sum  OutDataType=fixdt(1, 16)  OutScaling=2^-10
  Add2 : Sum  OutDataType=fixdt(1, 16)  OutScaling=2^-10
  I : dspmtrx3/Constant Diagonal Matrix  SystemSampleTime=-1  q=[1 1 1 ]  frame=off  dataType=Inherit from 'Constant(s) along diagonal'  isSigned=on  wordLen=16  udDataType=sfix(16)  fracBitsMode=Best precision  numFracBits=15
  Product : Product  Multiplication=Matrix(*)  OutDataType=fixdt(1, 16)  OutScaling=2^0  RndMeth=Zero
  Product1 : Product  OutDataType=fixdt(1, 16)  OutScaling=2^0  RndMeth=Zero
  Product2 : Product  Multiplication=Matrix(*)  OutDataType=fixdt(1, 16)  OutScaling=2^0  RndMeth=Zero
  Product3 : Product  Inputs=3  Multiplication=Matrix(*)  OutDataType=fixdt(1, 16)  OutScaling=2^0  RndMeth=Zero
  Product4 : Product  Multiplication=Matrix(*)  OutDataType=fixdt(1, 16)  OutScaling=2^0  RndMeth=Zero
  Subtract : Sum  Inputs=+-  OutDataType=fixdt(1, 16)  OutScaling=2^-10
  Sum : Sum  Inputs=-++  OutDataType=fixdt(1, 16)  OutScaling=2^-10
  sigma : Outport
  wires:
  Sum/1 -> sigma/1
  K_p/1 -> Subtract/1
  Product1/1 -> Subtract/2
  kappa1/1 -> Product1/1
  I/1 -> Product1/2
  S^T/1 -> Product/1, Product3/1
  z_1/1 -> Product/2
  Product/1 -> Add/1
  nu/1 -> Add/2
  Subtract/1 -> Product2/1
  Add/1 -> Product2/2
  Product2/1 -> Sum/1
  g_q/1 -> Add1/1
  g_s/1 -> Add1/2
  g_q^t/1 -> Add2/1
  g_s^t/1 -> Add2/2
  R^T/1 -> Product3/2, Product4/1
  Add1/1 -> Product3/3
  Add2/1 -> Product4/2
  Product3/1 -> Sum/2
  Product4/1 -> Sum/3

== system CSE1_CV3_1Straight/Control Systems/LgV design 2/z_1 eq ==
  eta : Inport
  chi : Inport  Port=2
  R^T : Inport  Port=3
  Product : Product  Multiplication=Matrix(*)  OutDataType=fixdt(1, 16)  OutScaling=2^0  RndMeth=Zero
  Subtract : Sum  Inputs=+-  OutDataType=fixdt(1, 16)  OutScaling=2^-10
  heading to pipi : Subsystem
  heading to pipi1 : Subsystem
  z_1 : Outport
  wires:
  R^T/1 -> Product/1
  eta/1 -> heading to pipi/1(In1)
  chi/1 -> Subtract/2
  Subtract/1 -> heading to pipi1/1(In1)
  Product/1 -> z_1/1
  heading to pipi/1(Out1) -> Subtract/1
  heading to pipi1/1(Out1) -> Product/2

== system CSE1_CV3_1Straight/Control Systems/LgV design 2/z_2 eq ==
  nu : Inport
  alpha : Inport  Port=2
  Subtract : Sum  Inputs=+-  OutDataType=fixdt(1, 16)  OutScaling=2^-10
  z_2 : Outport
  wires:
  nu/1 -> Subtract/1
  alpha/1 -> Subtract/2
  Subtract/1 -> z_2/1

== system CSE1_CV3_1Straight/Control Systems/Manual Thruster control/Subsystem ==
  u_act : Inport  OutDataType=fixdt(1, 16)  OutScaling=2^0
  Bus Selector : BusSelector  OutputSignals=u_1,u_2,u_3,u_4,u_5
  Mux : Mux  Inputs=5
  f_act to tau : Subsystem
  u_act to f_act : Subsystem
  tau : Outport
  wires:
  u_act/1 -> Bus Selector/1
  f_act to tau/1(tau) -> tau/1
  u_act to f_act/1(f_act) -> f_act to tau/1(f_act)
  Mux/1 -> u_act to f_act/1(u_act)
  Bus Selector/1 -> Mux/1  "<u_1>"
  Bus Selector/2 -> Mux/2  "<u_2>"
  Bus Selector/3 -> Mux/3  "<u_3>"
  Bus Selector/4 -> Mux/4  "<u_4>"
  Bus Selector/5 -> Mux/5  "<u_5>"

== system CSE1_CV3_1Straight/Control Systems/Nonlinear PID/Auxilary functions g_q ==
  f_q : Inport
  psi_los^q : Inport  Port=2
  f_q^q : Inport  Port=3
  psi_los^q^2 : Inport  Port=4
  f_q^s : Inport  Port=5
  psi_los^qs : Inport  Port=6
  f_q^t : Inport  Port=7
  g_q eq : Subsystem
  g_q^q eq : Subsystem
  g_q^s eq : Subsystem
  g_q^t eq : Subsystem
  g_q^q : Outport
  g_q^s : Outport  Port=2
  g_q^t : Outport  Port=3
  g_q : Outport  Port=4
  wires:
  g_q eq/1(g_q) -> g_q/1
  psi_los^q/1 -> g_q^q eq/2(psi_los^q), g_q^s eq/2(psi_los^q), g_q^t eq/1(psi_los^q), g_q eq/2(psi_los^q)
  f_q/1 -> g_q^q eq/1(f_q), g_q^s eq/1(f_q), g_q eq/1(f_q)
  f_q^q/1 -> g_q^q eq/3(f_q^q)
  psi_los^q^2/1 -> g_q^q eq/4(psi_los^q^2)
  g_q^q eq/1(g_q^q) -> g_q^q/1
  g_q^s eq/1(g_q^s) -> g_q^s/1
  f_q^s/1 -> g_q^s eq/3(f_q^s)
  psi_los^qs/1 -> g_q^s eq/4(psi_los^qs)
  g_q^t eq/1(g_q^t) -> g_q^t/1
  f_q^t/1 -> g_q^t eq/2(f_q^t)

== system CSE1_CV3_1Straight/Control Systems/Nonlinear PID/Auxiliary function g_s ==
  psi_los^sq : Inport
  f_s : Inport  Port=2
  psi_los^s : Inport  Port=3
  f_s^q : Inport  Port=4
  f_s^s : Inport  Port=5
  psi_los^s^2 : Inport  Port=6
  f_s^t : Inport  Port=7
  g_s eq : Subsystem
  g_s^q eq : Subsystem
  g_s^s eq : Subsystem
  g_s^t eq : Subsystem
  g_s^q : Outport
  g_s^s : Outport  Port=2
  g_s^t : Outport  Port=3
  g_s : Outport  Port=4
  wires:
  f_s/1 -> g_s eq/1(f_s), g_s^q eq/1(f_s), g_s^s eq/1(f_s)
  psi_los^s/1 -> g_s eq/2(psi_los^s), g_s^q eq/2(psi_los^s), g_s^s eq/2(psi_los^s), g_s^t eq/1(psi_los^s)
  g_s eq/1(g_s) -> g_s/1
  f_s^q/1 -> g_s^q eq/3(f_s^q)
  psi_los^sq/1 -> g_s^q eq/4(psi_los^sq)
  g_s^q eq/1(g_s^q) -> g_s^q/1
  g_s^s eq/1(g_s^s) -> g_s^s/1
  f_s^s/1 -> g_s^s eq/3(f_s^s)
  psi_los^s^2/1 -> g_s^s eq/4(psi_los^s^2)
  g_s^t eq/1(g_a^t) -> g_s^t/1
  f_s^t/1 -> g_s^t eq/2(f_s^t)

== system CSE1_CV3_1Straight/Control Systems/Nonlinear PID/Control law ==
  e : Inport
  a_d : Inport  Port=2
  v_d : Inport  Port=3
  nu : Inport  Port=4
  nu tilde : Inport  Port=5
  R^T : Inport  Port=6
  zeta : Inport  Port=7
  K_p : Inport  Port=8
  K_i : Inport  Port=9
  K_d : Inport  Port=10
  S(r) : Subsystem
  Sum : Sum  Inputs=+++  OutDataType=fixdt(1, 16)  OutScaling=2^-10
  r : Selector  InputPortWidth=3  IndexOptions=Index vector (dialog)  Indices=[3]  OutputSizes=1
  tau_FF : Subsystem
  tau_FL : Subsystem
  tau_PID : Subsystem
  tau : Outport
  wires:
  Sum/1 -> tau/1
  tau_PID/1(tau_PID) -> Sum/1
  K_p/1 -> tau_PID/2(K_p)
  R^T/1 -> tau_PID/1(R^T), tau_FF/4(R^T)
  K_i/1 -> tau_PID/4(K_i)
  zeta/1 -> tau_PID/5(zeta)
  K_d/1 -> tau_PID/6(K_d)
  nu/1 -> tau_FL/1(nu), r/1
  tau_FL/1(tau_FL) -> Sum/2
  r/1 -> S(r)/1(r)
  tau_FF/1(tau_FF) -> Sum/3
  e/1 -> tau_PID/3(e)
  nu tilde/1 -> tau_PID/7(nu tilde)
  S(r)/1(S) -> tau_FF/1(S)
  a_d/1 -> tau_FF/2(a_d)
  v_d/1 -> tau_FF/3(v_d)

== system CSE1_CV3_1Straight/Control Systems/Nonlinear PID/Error ==
  eta : Inport
  chi : Inport  Port=2
  Subtract : Sum  Inputs=+-  OutDataType=fixdt(1, 16)  OutScaling=2^-10
  heading to pipi : Subsystem
  heading to pipi1 : Subsystem
  e : Outport
  wires:
  chi/1 -> Subtract/2
  Subtract/1 -> heading to pipi1/1(In1)
  eta/1 -> heading to pipi/1(In1)
  heading to pipi1/1(Out1) -> e/1
  heading to pipi/1(Out1) -> Subtract/1

== system CSE1_CV3_1Straight/Control Systems/Nonlinear PID/Gamma_q ==
  11 : Inport
  22 : Inport  Port=2
  12 : Constant  Value=0
  21 : Constant  Value=0
  2x2 : Reshape  OutputDimensionality=Customize  OutputDimensions=[2,2]
  Mux : Mux
  Gamma_q : Outport
  wires:
  2x2/1 -> Gamma_q/1
  Mux/1 -> 2x2/1
  11/1 -> Mux/1
  21/1 -> Mux/2
  12/1 -> Mux/3
  22/1 -> Mux/4

== system CSE1_CV3_1Straight/Control Systems/Nonlinear PID/Integral action state ==
  nu tilde : Inport
  R : Inport  Port=2
  Product : Product  Multiplication=Matrix(*)  OutDataType=fixdt(1, 16)  OutScaling=2^0  RndMeth=Zero
  dot zeta : Outport
  wires:
  Product/1 -> dot zeta/1
  R/1 -> Product/1
  nu tilde/1 -> Product/2

== system CSE1_CV3_1Straight/Control Systems/Nonlinear PID/K_d ==
  11 : Inport
  22 : Inport  Port=2
  33 : Inport  Port=3
  {12..13,21,23,31..32} (6 alike) : Constant  Value=0
  Mux : Mux  Inputs=9
  R(psi) : Reshape  OutputDimensionality=Customize  OutputDimensions=[3,3]
  K_d : Outport
  wires:
  R(psi)/1 -> K_d/1
  Mux/1 -> R(psi)/1
  11/1 -> Mux/1
  21/1 -> Mux/2
  31/1 -> Mux/3
  12/1 -> Mux/4
  22/1 -> Mux/5
  32/1 -> Mux/6
  13/1 -> Mux/7
  23/1 -> Mux/8
  33/1 -> Mux/9

== system CSE1_CV3_1Straight/Control Systems/Nonlinear PID/K_i ==
  11 : Inport
  22 : Inport  Port=2
  33 : Inport  Port=3
  {12..13,21,23,31..32} (6 alike) : Constant  Value=0
  Mux : Mux  Inputs=9
  R(psi) : Reshape  OutputDimensionality=Customize  OutputDimensions=[3,3]
  K_i : Outport
  wires:
  R(psi)/1 -> K_i/1
  Mux/1 -> R(psi)/1
  11/1 -> Mux/1
  21/1 -> Mux/2
  31/1 -> Mux/3
  12/1 -> Mux/4
  22/1 -> Mux/5
  32/1 -> Mux/6
  13/1 -> Mux/7
  23/1 -> Mux/8
  33/1 -> Mux/9

== system CSE1_CV3_1Straight/Control Systems/Nonlinear PID/K_p ==
  11 : Inport
  22 : Inport  Port=2
  33 : Inport  Port=3
  {12..13,21,23,31..32} (6 alike) : Constant  Value=0
  Mux : Mux  Inputs=9
  R(psi) : Reshape  OutputDimensionality=Customize  OutputDimensions=[3,3]
  K_p : Outport
  wires:
  R(psi)/1 -> K_p/1
  Mux/1 -> R(psi)/1
  11/1 -> Mux/1
  21/1 -> Mux/2
  31/1 -> Mux/3
  12/1 -> Mux/4
  22/1 -> Mux/5
  32/1 -> Mux/6
  13/1 -> Mux/7
  23/1 -> Mux/8
  33/1 -> Mux/9

== system CSE1_CV3_1Straight/Control Systems/Nonlinear PID/R(psi) ==
  psi : Inport
  Mux : Mux  Inputs=9
  R(psi) : Reshape  OutputDimensionality=Customize  OutputDimensions=[3,3]
  R11 : Fcn  Expr=cos(u(1))
  R12 : Fcn  Expr=-1*sin(u(1))
  R{13,23,31..32} (4 alike) : Constant  Value=0
  R21 : Fcn  Expr=sin(u(1))
  R22 : Fcn  Expr=cos(u(1))
  R33 : Constant
  R : Outport
  wires:
  R(psi)/1 -> R/1
  Mux/1 -> R(psi)/1
  psi/1 -> R11/1, R21/1, R12/1, R22/1
  R11/1 -> Mux/1
  R21/1 -> Mux/2
  R31/1 -> Mux/3
  R12/1 -> Mux/4
  R22/1 -> Mux/5
  R32/1 -> Mux/6
  R13/1 -> Mux/7
  R33/1 -> Mux/9
  R23/1 -> Mux/8

== system CSE1_CV3_1Straight/Control Systems/Nonlinear PID/Thruster allocation ==
  tau : Inport
  f_act to u_act : Subsystem
  tau to f_act : Subsystem
  u_act : Outport
  wires:
  tau/1 -> tau to f_act/1(tau)
  tau to f_act/1(f_act) -> f_act to u_act/1(f_act)
  f_act to u_act/1(u_act) -> u_act/1

== system CSE1_CV3_1Straight/Control Systems/Nonlinear PID/Update laws ==
  e : Inport
  chi^q : Inport  Port=2
  Gamma_q : Inport  Port=3
  lambda : Inport  Port=4
  K_p : Inport  Port=5
  f_s : Inport  Port=6
  f_q : Inport  Port=7
  Add : Sum  OutDataType=fixdt(1, 16)  OutScaling=2^-10
  Integrator : Integrator  ExternalReset=level  InitialConditionSource=external
  Integrator1 : Integrator  ExternalReset=level  InitialConditionSource=external  InitialCondition=250
  Product1 : Product  OutDataType=fixdt(1, 16)  OutScaling=2^0  RndMeth=Zero
  Product2 : Product  Inputs=3  Multiplication=Matrix(*)  OutDataType=fixdt(1, 16)  OutScaling=2^0  RndMeth=Zero
  Product3 : Product  Multiplication=Matrix(*)  OutDataType=fixdt(1, 16)  OutScaling=2^0  RndMeth=Zero
  Reset q : Constant  Value=0
  Reset s : Constant  Value=0
  Subtract : Sum  Inputs=+-  OutDataType=fixdt(1, 16)  OutScaling=2^-10
  Transpose : dspmtrx3/Transpose  SystemSampleTime=-1  Hermitian=off  overflowFlag=off
  dot omega_q : Gain  Gain=-1  ParameterDataType=fixdt(1, 16)  ParameterScaling=2^0  OutDataType=fixdt(1, 16)  OutScaling=2^0
  omega_q : Integrator
  q_0 : Subsystem
  s_0 : Constant  Value=0
  q : Outport  PortDimensions=2
  s : Outport  Port=2  PortDimensions=1
  dot q : Outport  Port=3  PortDimensions=2
  dot s : Outport  Port=4  PortDimensions=1
  wires:
  f_q/1 -> Add/2
  Add/1 -> Integrator/1, dot q/1
  chi^q/1 -> Transpose/1
  lambda/1 -> Product1/1
  Subtract/1 -> Product1/2
  Product1/1 -> dot omega_q/1
  dot omega_q/1 -> omega_q/1
  f_s/1 -> Integrator1/1, dot s/1
  Integrator/1 -> q/1
  Integrator1/1 -> s/1
  e/1 -> Product2/3
  Transpose/1 -> Product2/1
  K_p/1 -> Product2/2
  Gamma_q/1 -> Product3/1
  Product3/1 -> Subtract/2
  Product2/1 -> Product3/2
  omega_q/1 -> Add/1, Subtract/1
  Reset q/1 -> Integrator/2
  q_0/1(q_0) -> Integrator/3
  Reset s/1 -> Integrator1/2
  s_0/1 -> Integrator1/3

== system CSE1_CV3_1Straight/Control Systems/Nonlinear PID/a_d ==
  dot q : Inport
  dot s : Inport  Port=2
  g_q^q : Inport  Port=3
  g_q^s : Inport  Port=4
  g_q^t : Inport  Port=5
  g_s^q : Inport  Port=6
  g_s^s : Inport  Port=7
  g_s^t : Inport  Port=8
  Product : Product  Multiplication=Matrix(*)  OutDataType=fixdt(1, 16)  OutScaling=2^0  RndMeth=Zero
  Product1 : Product  Multiplication=Matrix(*)  OutDataType=fixdt(1, 16)  OutScaling=2^0  RndMeth=Zero
  Sum : Sum  Inputs=+++  OutDataType=fixdt(1, 16)  OutScaling=2^-10
  v_d^q : Subsystem
  v_d^s : Subsystem
  v_d^t : Subsystem
  a_d : Outport
  wires:
  g_q^q/1 -> v_d^q/1(g_q^q)
  g_s^q/1 -> v_d^q/2(g_s^q)
  Sum/1 -> a_d/1
  v_d^q/1(v_d^q) -> Product/1
  dot q/1 -> Product/2
  Product/1 -> Sum/1
  g_q^s/1 -> v_d^s/1(g_q^s)
  g_s^s/1 -> v_d^s/2(g_s^s)
  v_d^s/1(v_d^s) -> Product1/1
  dot s/1 -> Product1/2
  g_q^t/1 -> v_d^t/1(g_q^t)
  g_s^t/1 -> v_d^t/2(g_s^t)
  Product1/1 -> Sum/2
  v_d^t/1(v_d^t) -> Sum/3

== system CSE1_CV3_1Straight/Control Systems/Nonlinear PID/nu tilde ==
  nu : Inport
  v_d : Inport  Port=2
  R^T : Inport  Port=3
  Product : Product  Multiplication=Matrix(*)  OutDataType=fixdt(1, 16)  OutScaling=2^0  RndMeth=Zero
  Subtract : Sum  Inputs=+-  OutDataType=fixdt(1, 16)  OutScaling=2^-10
  nu tilde : Outport
  wires:
  nu/1 -> Subtract/1
  Product/1 -> Subtract/2
  R^T/1 -> Product/1
  v_d/1 -> Product/2
  Subtract/1 -> nu tilde/1

== system CSE1_CV3_1Straight/Control Systems/Nonlinear PID/v_d ==
  g_q : Inport
  g_s : Inport  Port=2
  Add : Sum  OutDataType=fixdt(1, 16)  OutScaling=2^-10
  v_d : Outport
  wires:
  g_q/1 -> Add/1
  g_s/1 -> Add/2
  Add/1 -> v_d/1

== system CSE1_CV3_1Straight/Control Systems/Precision control/Subsystem ==
  u_act : Inport  OutDataType=fixdt(1, 16)  OutScaling=2^0
  Bus Selector : BusSelector  OutputSignals=signal1,signal2,signal3,signal4,signal5
  Mux : Mux  Inputs=5
  f_act to tau : Subsystem
  u_act to f_act : Subsystem
  tau : Outport
  wires:
  u_act/1 -> Bus Selector/1
  f_act to tau/1(tau) -> tau/1
  u_act to f_act/1(f_act) -> f_act to tau/1(f_act)
  Mux/1 -> u_act to f_act/1(u_act)
  Bus Selector/1 -> Mux/1  "<signal1>"
  Bus Selector/2 -> Mux/2  "<signal2>"
  Bus Selector/3 -> Mux/3  "<signal3>"
  Bus Selector/4 -> Mux/4  "<signal4>"
  Bus Selector/5 -> Mux/5  "<signal5>"

== system CSE1_CV3_1Straight/Control Systems/Simple Control/Thruster allocation ==
  tau : Inport
  f_act to u_act : Subsystem
  tau to f_act : Subsystem
  u_act : Outport
  wires:
  tau/1 -> tau to f_act/1(tau)
  tau to f_act/1(f_act) -> f_act to u_act/1(f_act)
  f_act to u_act/1(u_act) -> u_act/1

== system CSE1_CV3_1Straight/Guidance Systems/Path-following/Heading ==
  p_d^s : Inport
  p_d^s^2 : Inport  Port=2
  p_d^s^3 : Inport  Port=3
  Demux : Demux  Outputs=2
  Demux1 : Demux  Outputs=2
  Demux2 : Demux  Outputs=2
  psi_d eq : Subsystem
  psi_d^s eq : Subsystem
  psi_d^s^2 eq : Subsystem
  psi_d : Outport
  psi_d^s : Outport  Port=2
  psi_d^s^2 : Outport  Port=3
  wires:
  psi_d eq/1(psi_d) -> psi_d/1
  Demux/1 -> psi_d eq/1(x_d^s), psi_d^s eq/1(x_d^s), psi_d^s^2 eq/3(x_d^s)
  Demux/2 -> psi_d eq/2(y_d^s), psi_d^s eq/2(y_d^s), psi_d^s^2 eq/4(y_d^s)
  p_d^s/1 -> Demux/1
  p_d^s^2/1 -> Demux1/1
  Demux1/1 -> psi_d^s eq/3(x_d^s^2), psi_d^s^2 eq/5(x_d^s^2)
  Demux1/2 -> psi_d^s eq/4(y_d^s^2), psi_d^s^2 eq/6(y_d^s^2)
  psi_d^s eq/1(psi_d^s) -> psi_d^s/1
  p_d^s^3/1 -> Demux2/1
  psi_d^s^2 eq/1(psi_d^s^2) -> psi_d^s^2/1
  Demux2/1 -> psi_d^s^2 eq/7(x_d^s^3)
  Demux2/2 -> psi_d^s^2 eq/8(y_d^s^3)
  psi_d^s eq/2(num) -> psi_d^s^2 eq/1(num)
  psi_d^s eq/3(den) -> psi_d^s^2 eq/2(den)

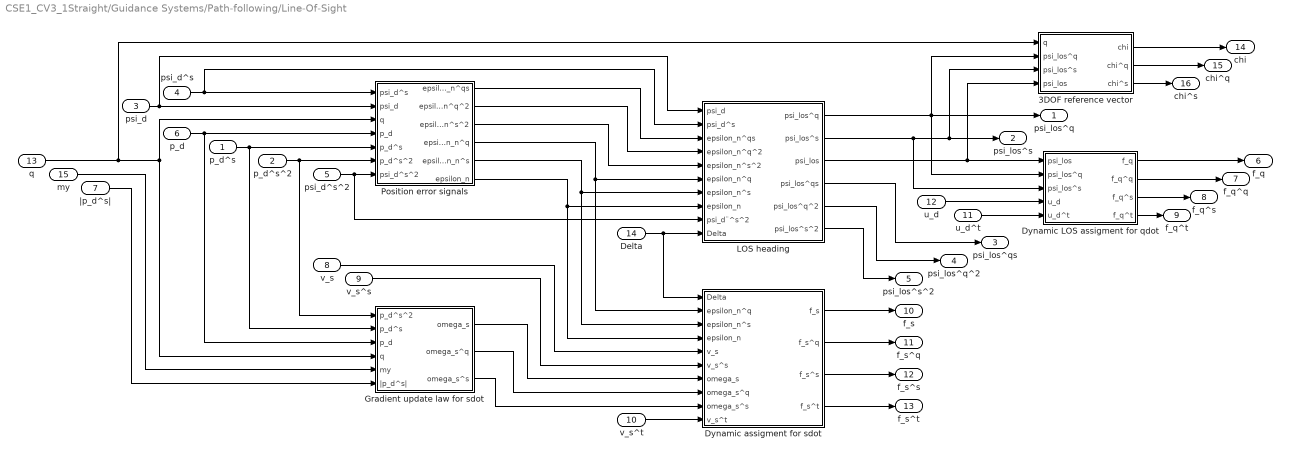
== system CSE1_CV3_1Straight/Guidance Systems/Path-following/Line-Of-Sight ==
  p_d^s : Inport
  p_d^s^2 : Inport  Port=2
  psi_d : Inport  Port=3
  psi_d^s : Inport  Port=4
  psi_d^s^2 : Inport  Port=5
  p_d : Inport  Port=6
  |p_d^s| : Inport  Port=7
  v_s : Inport  Port=8
  v_s^s : Inport  Port=9
  v_s^t : Inport  Port=10
  u_d^t : Inport  Port=11
  u_d : Inport  Port=12
  q : Inport  Port=13
  Delta : Inport  Port=14
  my : Inport  Port=15
  3DOF reference vector : Subsystem
  Dynamic LOS assigment for qdot : Subsystem
  Dynamic assigment for sdot : Subsystem
  Gradient update law for sdot : Subsystem
  LOS heading : Subsystem
  Position error signals : Subsystem
  psi_los^q : Outport
  psi_los^s : Outport  Port=2
  psi_los^qs : Outport  Port=3
  psi_los^q^2 : Outport  Port=4
  psi_los^s^2 : Outport  Port=5
  f_q : Outport  Port=6
  "f_q^q " : Outport  Port=7
  f_q^s : Outport  Port=8
  f_q^t : Outport  Port=9
  f_s : Outport  Port=10
  f_s^q : Outport  Port=11
  f_s^s : Outport  Port=12
  f_s^t : Outport  Port=13
  chi : Outport  Port=14
  chi^q : Outport  Port=15
  chi^s : Outport  Port=16
  wires:
  Dynamic assigment for sdot/1(f_s) -> f_s/1
  Delta/1 -> Dynamic assigment for sdot/1(Delta), LOS heading/10(Delta)
  psi_d/1 -> Position error signals/2(psi_d), LOS heading/1(psi_d)
  v_s/1 -> Dynamic assigment for sdot/5(v_s)
  Gradient update law for sdot/1(omega_s) -> Dynamic assigment for sdot/7(omega_s)
  p_d^s/1 -> Gradient update law for sdot/2(p_d^s), Position error signals/5(p_d^s)
  my/1 -> Gradient update law for sdot/5(my)
  |p_d^s|/1 -> Gradient update law for sdot/6(|p_d^s|)
  u_d/1 -> Dynamic LOS assigment for qdot/4(u_d)
  LOS heading/3(psi_los) -> Dynamic LOS assigment for qdot/1(psi_los), 3DOF reference vector/4(psi_los)
  p_d/1 -> Position error signals/4(p_d), Gradient update law for sdot/3(p_d)
  q/1 -> Position error signals/3(q), Gradient update law for sdot/4(q), 3DOF reference vector/1(q)
  Position error signals/6(epsilon_n) -> Dynamic assigment for sdot/4(epsilon_n), LOS heading/8(epsilon_n)
  Position error signals/5(epsilon_n^s) -> LOS heading/7(epsilon_n^s), Dynamic assigment for sdot/3(epsilon_n^s)
  Position error signals/1(epsilon_n^qs) -> LOS heading/3(epsilon_n^qs)
  Position error signals/2(epsilon_n^q^2) -> LOS heading/4(epsilon_n^q^2)
  Position error signals/3(epsilon_n^s^2) -> LOS heading/5(epsilon_n^s^2)
  psi_d^s/1 -> Position error signals/1(psi_d^s), LOS heading/2(psi_d^s)
  Position error signals/4(epsilon_n^q) -> LOS heading/6(epsilon_n^q), Dynamic assigment for sdot/2(epsilon_n^q)
  LOS heading/1(psi_los^q) -> 3DOF reference vector/2(psi_los^q), Dynamic LOS assigment for qdot/2(psi_los^q), psi_los^q/1
  LOS heading/2(psi_los^s) -> Dynamic LOS assigment for qdot/3(psi_los^s), 3DOF reference vector/3(psi_los^s), psi_los^s/1
  3DOF reference vector/1(chi) -> chi/1
  3DOF reference vector/2(chi^q) -> chi^q/1
  3DOF reference vector/3(chi^s) -> chi^s/1
  Dynamic LOS assigment for qdot/2("f_q^q ") -> "f_q^q "/1
  Dynamic LOS assigment for qdot/3(f_q^s) -> f_q^s/1
  Dynamic LOS assigment for qdot/4(f_q^t) -> f_q^t/1
  p_d^s^2/1 -> Position error signals/6(p_d^s^2), Gradient update law for sdot/1(p_d^s^2)
  Dynamic LOS assigment for qdot/1(f_q) -> f_q/1
  v_s^s/1 -> Dynamic assigment for sdot/6(v_s^s)
  Gradient update law for sdot/2(omega_s^q) -> Dynamic assigment for sdot/8(omega_s^q)
  Gradient update law for sdot/3(omega_s^s) -> Dynamic assigment for sdot/9(omega_s^s)
  psi_d^s^2/1 -> Position error signals/7(psi_d^s^2), LOS heading/9(psi_d¨^s^2)
  Dynamic assigment for sdot/4(f_s^t) -> f_s^t/1
  Dynamic assigment for sdot/3(f_s^s) -> f_s^s/1
  Dynamic assigment for sdot/2(f_s^q) -> f_s^q/1
  LOS heading/4(psi_los^qs) -> psi_los^qs/1
  LOS heading/5(psi_los^q^2) -> psi_los^q^2/1
  LOS heading/6(psi_los^s^2) -> psi_los^s^2/1
  u_d^t/1 -> Dynamic LOS assigment for qdot/5(u_d^t)
  v_s^t/1 -> Dynamic assigment for sdot/10(v_s^t)

== system CSE1_CV3_1Straight/Guidance Systems/Path-following/Path ==
  s : Inport
  x_1 : Inport  Port=2
  y_1 : Inport  Port=3
  x_2 : Inport  Port=4
  y_2 : Inport  Port=5
  Straight path : Subsystem
  p_d^s : Outport
  p_d^s^2 : Outport  Port=2
  p_d^s^3 : Outport  Port=3
  p_d : Outport  Port=4
  |p_d^s| : Outport  Port=5
  wires:
  s/1 -> Straight path/1(s)
  x_2/1 -> Straight path/4(x_2)
  y_2/1 -> Straight path/5(y_2)
  x_1/1 -> Straight path/2(x_1)
  y_1/1 -> Straight path/3(y1)
  Straight path/1(p_d) -> p_d/1  "p_d"
  Straight path/2(p_d^s) -> p_d^s/1  "p_d^s"
  Straight path/3(p_d^s^2) -> p_d^s^2/1  "p_d^s^2"
  Straight path/4(p_d^s^3) -> p_d^s^3/1  "p_d^s^3"
  Straight path/5(|p_d^s|) -> |p_d^s|/1  "|p_d^s|"

== system CSE1_CV3_1Straight/Guidance Systems/Path-following/Speed assigment ==
  |p_d^s| : Inport
  p_d^s : Inport  Port=2
  p_d^s^2 : Inport  Port=3
  u_d : Inport  Port=4
  Derivative : Derivative
  v_s eq : Subsystem
  v_s^s eq : Subsystem
  v_s^t eq : Subsystem
  v_s : Outport
  v_s^s : Outport  Port=2
  v_s^t : Outport  Port=3
  u_d^t : Outport  Port=4
  wires:
  v_s eq/1(v_s) -> v_s/1
  |p_d^s|/1 -> v_s eq/1(|p_d^s|), v_s^s eq/1(|p_d^s|), v_s^t eq/1(|p_d^s|)
  u_d/1 -> v_s eq/2(u_d), v_s^s eq/2(u_d), Derivative/1
  v_s^s eq/1(v_s^s) -> v_s^s/1
  p_d^s/1 -> v_s^s eq/3(p_d^s)
  p_d^s^2/1 -> v_s^s eq/4(p_d^s^2)
  v_s^t eq/1(v_s^t) -> v_s^t/1
  Derivative/1 -> v_s^t eq/2(u_d^t), u_d^t/1

== system CSE1_CV3_1Straight/Plants/CSE1/Bow Thruster ==
  Bow Thruster Direction u_5 : Inport
  Bow Thruster Power : Inport  Port=2
  Add : Sum  Inputs=+++
  BT_D_Gain1 : Gain  Gain=0.02
  BT_D_Gain2 : Gain  Gain=0.02
  BT_L_Gain1 : Gain  Gain=0.02
  BT_L_Gain2 : Gain  Gain=-0.02
  BT_Power_Offset1 : Constant  Value=0.05
  BT_Power_Offset2 : Constant  Value=0.05
  BT_Power_Offset3 : Constant  Value=0.05
  Constant : Constant  Value=0  OutDataType=fixdt(1, 16)  OutScaling=2^0
  Constant1 : Constant  Value=0  OutDataType=fixdt(1, 16)  OutScaling=2^0
  Neg : Gain  Gain=-1  ParameterDataType=fixdt(1, 16)  ParameterScaling=2^0  OutDataType=fixdt(1, 16)  OutScaling=2^0
  SIT Out5 BT : S-Function  Priority=1  FunctionName=NI_SIT_IO  Parameters=width dtype portnum stime stype btype  EnableBusSupport=off  mask(SIT Outport){portnum=1, width=-1, stime=-1, dtype=auto, stype=auto, btype=0}
      mask prompts: portnum "Port number:"; width "Port dimensions (-1 for dynamically sized):"; stime "Sample time (-1 for inherited):"; dtype "Data type:"; stype "Signal type:"; btype "Block type:"
      mask help: Use this outport on any level of nested subsystems to allow the LabVIEW Simulation Interface Toolkit to map hardware to it.
      mask init:
      | NI_SIT_IO_init;
      settings: CopyFcn=NI_SIT_IO_callbacks(1);  DeleteFcn=NI_SIT_IO_callbacks(2);
      mask StyleString: edit,edit,edit,popup(auto|double|single|int8|uint8|int16|uint16|int32|uint32|boolean),popup(auto|real|complex),edit
      mask CallbackString: NI_SIT_IO_callbacks(3);|||NI_SIT_IO_callbacks(4);||
      mask TabNameString: Parameters,Parameters,Parameters,Parameters,Parameters,Parameters
      mask Display:
      | patch([-x x], [-y y], [.90980 .81960 .32156]);
      | plot([0 -x x 0], [rad -y y rad]);
      | fprintf('SIT%d', portnum);
  Saturation Dynamic : simulink/Discontinuities/Saturation Dynamic  SystemSampleTime=-1  OutMin=[]  OutMax=[]  OutDataTypeStr=Inherit: Same as second input  OutDataType=fixdt(1, 16)  OutScaling=2^-10  DoSatur=off
  Saturation Dynamic1 : simulink/Discontinuities/Saturation Dynamic  SystemSampleTime=-1  OutMin=[]  OutMax=[]  OutDataTypeStr=Inherit: Same as second input  OutDataType=fixdt(1, 16)  OutScaling=2^-10  DoSatur=off
  Saturation Dynamic2 : simulink/Discontinuities/Saturation Dynamic  SystemSampleTime=-1  OutMin=[]  OutMax=[]  OutDataTypeStr=Inherit: Same as second input  OutDataType=fixdt(1, 16)  OutScaling=2^-10  DoSatur=off
  Sum1 : Sum  Inputs=|++
  Sum2 : Sum  Inputs=|++
  Terminator : Terminator
  Terminator1 : Terminator
  wires:
  Bow Thruster Direction u_5/1 -> BT_D_Gain1/1, Saturation Dynamic1/2, BT_D_Gain2/1, Saturation Dynamic2/2
  BT_D_Gain1/1 -> Add/1
  BT_D_Gain2/1 -> Add/3
  BT_Power_Offset1/1 -> Add/2
  Add/1 -> Saturation Dynamic/2
  Bow Thruster Power/1 -> BT_L_Gain2/1, Saturation Dynamic2/1, BT_L_Gain1/1, Neg/1
  Sum1/1 -> Saturation Dynamic/1
  BT_L_Gain1/1 -> Sum1/1
  BT_L_Gain2/1 -> Sum2/1
  Sum2/1 -> Saturation Dynamic/3
  BT_Power_Offset2/1 -> Sum1/2
  BT_Power_Offset3/1 -> Sum2/2
  Saturation Dynamic/1 -> SIT Out5 BT/1
  Saturation Dynamic2/1 -> Terminator1/1
  Saturation Dynamic1/1 -> Terminator/1
  Constant/1 -> Saturation Dynamic1/1
  Constant1/1 -> Saturation Dynamic2/3
  Neg/1 -> Saturation Dynamic1/3
